simulink model "FullCardioLabModel"  (R2023b)
settings: Solver=FixedStepDiscrete  StartTime=0.0  StopTime=param_sim_time  FixedStep=1/fs  MaxStep=1/fs  RelTol=1e-3
undefined symbols (not defined in the file): analyses, fdesignblkfcn, fs, gcbh, param_tot_samples
libraries: dspstat3 x13, SCGAnalysis_SignalGenerationLib x2
(part 13 of 20)

== matlab function FullCardioLabModel/SCG Analysis/Enabled SCG Analysis Subsystem/Cardiac Interval Identification/Systolic Fiducial Point Marker/3D Systolic Fiducial Point Identifier ==
  data: fs input size=[1]; MC output size=[4*ceil(param_sim_time) 1]; MC_prelim input; IM_prelim input; IM output size=[4*ceil(param_sim_time) 1]; AO output size=[4*ceil(param_sim_time) 1]; AO_prelim input; scg_s1_3DMod input
function [MC, IM, AO] = slk_3D_systolic_fiducial_point_identifier(fs, MC_prelim, IM_prelim, AO_prelim, scg_s1_3DMod)
% Function to identify the (final) systolic hemodynamic fiducial points of the seismocardiogram (SCG) based on the preliminary systolic markers and using an S1 3D modulus signal.

% INPUTS:
% fs - the sampling frequency (in Hz).
% MC_prelim - preliminary sample indexes of mitral closure.
% IM_prelim - preliminary sample indexes isovolumic moment.
% AO_prelim_ - preliminary sample indexes of aortic opening.
% scg_s1_3DMod - the systolic (i.e, constructed from the S1 bandwidth-optimized x,y,z SCG components) 3DModulus signal.

% OUTPUTS:
% MC - final sample indexes of mitral closure.
% IM - final sample indexes isovolumic moment.
% AO - final sample indexes of aortic opening.

coder.extrinsic('legend');

% Plotting before refining.
Labelled3DSCG = figure;
plot(scg_s1_3DMod); hold on;
plot(IM_prelim, scg_s1_3DMod(IM_prelim),'xr')
plot(MC_prelim, scg_s1_3DMod(MC_prelim),'xb')
plot(AO_prelim, scg_s1_3DMod(AO_prelim),'xk')
box off

title('Systolic Fiducial Markers')
xlabel('Sample no.')
ylabel('Acceleration (mg)')

IM = zeros(length(IM_prelim), 1);   % Pre-initalization for speed.
MC = zeros(length(MC_prelim), 1);
AO = zeros(length(AO_prelim), 1);

MC_search_window_size = fs*0.02; % The window centered about MC_prelim where we will search for MC in the 3D Mod signal.
IM_search_window_size = fs*0.02; % The window centered about MC_prelim where we will search for MC in the 3D Mod signal.
AO_search_window_size = fs*0.04; % The window centered about MC_prelim where we will search for MC in the 3D Mod signal.


% Refining MC
for i = 1:length(MC_prelim)
    
    MC_search_window = scg_s1_3DMod(MC_prelim(i) - floor(MC_search_window_size/2):MC_prelim(i) + ceil(MC_search_window_size/2));
    [MC_candies_amps, MC_candies_locs, MC_candies_widths, MC_candies_proms]  = findpeaks(MC_search_window); % Identifying the amplitude, location, width, and prominence of the detected peaks.
    
    if MC_candies_amps % If peaks were detected...
        %MC_candy = MC_candies_locs(find(MC_candies_amps == max(MC_candies_amps))); % Consider MC as the peak with the maximum amplitude.
        %MC_candy = MC_candies_locs(1); % Consider MC as the first peak
        %MC_candy = MC_candies_locs(find(MC_candies_widths == max(MC_candies_widths))); % Consider MC as the peak with the greatest width.
        MC_candy = MC_candies_locs(find(MC_candies_proms == max(MC_candies_proms))); % Consider MC as the peak with the maximum prominence.
        MC(i) = -1 + MC_prelim(i) - floor(MC_search_window_size/2) + MC_candy;
    else
        MC(i) = nan;
    end
    
    MC_candy = []; % Clearing.
    MC_candies_amps = [];
    MC_candies_locs = [];
    MC_candies_widths = [];
    MC_candies_proms = [];
    
end

% Refining IM
for i = 1:length(IM_prelim)
    
    IM_search_window = scg_s1_3DMod(IM_prelim(i) - floor(IM_search_window_size/2):IM_prelim(i) + ceil(IM_search_window_size/2));
    [IM_candies_amps, IM_candies_locs, IM_candies_widths, IM_candies_proms]  = findpeaks(IM_search_window); % Identifying the amplitude, location, width, and prominence of the detected peaks.
    
    if IM_candies_amps % If peaks were detected...
        %IM_candy = IM_candies_locs(find(IM_candies_amps == max(IM_candies_amps))); % Consider IM as the peak with the maximum amplitude.
        %IM_candy = IM_candies_locs(1); % Consider IM as the first peak
        %IM_candy = IM_candies_locs(find(IM_candies_widths == max(IM_candies_widths))); % Consider IM as the peak with the greatest width.
        IM_candy = IM_candies_locs(find(IM_candies_proms == max(IM_candies_proms))); % Consider IM as the peak with the maximum prominence.
        IM(i) = -1 + IM_prelim(i) - floor(IM_search_window_size/2) + IM_candy;
    else
        IM(i) = nan;
    end
    
    IM_candy = []; % Clearing.
    IM_candies_amps = [];
    IM_candies_locs = [];
    IM_candies_widths = [];
    IM_candies_proms = [];
    
end

% Refining AO
for i = 1:length(AO_prelim)
    
    AO_lower_search_lim = max([IM(i), AO_prelim(i) - floor(AO_search_window_size/2)]); % Making sure the serach window does not include the IM peak.
    
    AO_search_window = scg_s1_3DMod(AO_lower_search_lim : AO_prelim(i) + ceil(AO_search_window_size/2));
    [AO_candies_amps, AO_candies_locs, AO_candies_widths, AO_candies_proms]  = findpeaks(AO_search_window); % Identifying the amplitude, location, width, and prominence of the detected peaks.
    
    if AO_candies_amps % If peaks were detected...
        %AO(i) = AO_candies_locs(find(AO_candies_amps == max(AO_candies_amps))); % Consider AO as the peak with the maximum amplitude.
        AO_candy = AO_candies_locs(1); % Consider AO as the first peak
        %AO_candy = AO_candies_locs(find(AO_candies_widths == max(AO_candies_widths))); % Consider AO as the peak with the greatest width.
        %AO_candy = AO_candies_locs(find(AO_candies_proms == max(AO_candies_proms))); % Consider AO as the peak with the maximum prominence.
        AO(i) = -1 + AO_lower_search_lim + AO_candy;
    else
        AO(i) = nan;
    end
    
    AO_candy = []; % Clearing.
    AO_candies_amps = [];
    AO_candies_locs = [];
    AO_candies_widths = [];
    AO_candies_proms = [];
    AO_lower_search_lim = [];
    
end

figure(Labelled3DSCG);
hold on;
plot(IM(~isnan(IM)), scg_s1_3DMod(IM(~isnan(IM))),'or') % Do not plot the 'nans'.
plot(MC(~isnan(MC)), scg_s1_3DMod(MC(~isnan(MC))),'ob')
plot(AO(~isnan(AO)), scg_s1_3DMod(AO(~isnan(AO))),'ok')

legend('3D Modulus','IM_p_r_e_l_i_m','MC_p_r_e_l_i_m','AO_p_r_e_l_i_m','IM','MC','AO')

end

== matlab function FullCardioLabModel/SCG Analysis/Enabled SCG Analysis Subsystem/Cardiac Interval Identification/Diastolic Fiducial Point Marker/3D Diastolic Fiducial Point Identifier ==
  data: fs input size=[1]; AC output size=[4*ceil(param_sim_time) 1]; AC_prelim input; MO_prelim input; MO output size=[4*ceil(param_sim_time) 1]; scg_s2_3DMod input
function [AC, MO] = slk_3D_diastolic_fiducial_point_identifier(fs, AC_prelim, MO_prelim, scg_s2_3DMod)
% Function to identify the (final) diastolic hemodynamic fiducial points of the seismocardiogram (SCG) based on the preliminary diastolic markers and using an S2 3D modulus signal.

% INPUTS:
% fs - the sampling frequency (in Hz).
% AC_prelim - preliminary sample indexes of aortic closure.
% MO_prelim - preliminary sample indexes mitral opening.
% scg_s2_3DMod - the diastolic (i.e, constructed from the S2 bandwidth-optimized x,y,z SCG components) 3DModulus signal.

% OUTPUTS:
% AC - final sample indexes of aortic opening.
% MO - final sample indexes of mitral opening.

coder.extrinsic('legend');

% Plotting before refining.
Labelled3DSCG = figure;
plot(scg_s2_3DMod); hold on;
plot(AC_prelim(~isnan(AC_prelim)), scg_s2_3DMod(AC_prelim(~isnan(AC_prelim))),'xb') % Do not plot the 'nans'.
plot(MO_prelim(~isnan(MO_prelim)), scg_s2_3DMod(MO_prelim(~isnan(MO_prelim))),'xr')
box off

title('Diastolic Fiducial Markers')
xlabel('Sample no.')
ylabel('Acceleration (mg)')

AC = zeros(length(MO_prelim), 1);   % Pre-initalization for speed.
MO = zeros(length(AC_prelim), 1);


AC_search_window_size = fs*0.02; % The window centered about AC_prelim where we will search for AC in the 3D Mod signal.
MO_search_window_size = fs*0.02; % The window centered about MO_prelim where we will search for MO in the 3D Mod signal.


% Refining AC
for i = 1:length(AC_prelim)
    
    if isnan(AC_prelim(i))
        
        AC(i) = nan;

    else
        
        AC_search_window = scg_s2_3DMod(AC_prelim(i) - floor(AC_search_window_size/2):AC_prelim(i) + ceil(AC_search_window_size/2));
        [AC_candies_amps, AC_candies_locs, AC_candies_widths, AC_candies_proms]  = findpeaks(AC_search_window); % Identifying the amplitude, location, width, and prominence of the detected peaks.
        
        if AC_candies_amps % If peaks were detected...
            %AC_candy = MC_candies_locs(find(MC_candies_amps == max(MC_candies_amps)));      % Consider AC as the peak with the maximum amplitude.
            %AC_candy = MC_candies_locs(1);                                                  % Consider AC as the first peak.
            %AC_candy = MC_candies_locs(find(MC_candies_widths == max(MC_candies_widths)));  % Consider AC as the peak with the greatest width.
            AC_candy = AC_candies_locs(find(AC_candies_proms == max(AC_candies_proms)));     % Consider AC as the peak with the maximum prominence.
            AC(i) = -1 + AC_prelim(i) - floor(AC_search_window_size/2) + AC_candy;
        else
            AC(i) = nan;
        end
        
        AC_candy = []; % Clearing.
        AC_candies_amps = [];
        AC_candies_locs = [];
        AC_candies_widths = [];
        AC_candies_proms = [];
        
    end
end

% Refining MO
for i = 1:length(MO_prelim)
    
    if isnan(MO_prelim(i))
        
        MO(i) = nan;
        
    else
        
        MO_search_window = scg_s2_3DMod(MO_prelim(i) - floor(MO_search_window_size/2):MO_prelim(i) + ceil(MO_search_window_size/2));
        [MO_candies_amps, MO_candies_locs, MO_candies_widths, MO_candies_proms]  = findpeaks(MO_search_window); % Identifying the amplitude, location, width, and prominence of the detected peaks.
        
        if MO_candies_amps % If peaks were detected...
            %MO_candy = IM_candies_locs(find(MO_candies_amps == max(MO_candies_amps)));       % Consider MO as the peak with the maximum amplitude.
            %MO_candy = IM_candies_locs(1);                                                   % Consider MO as the first peak
            %MO_candy = IM_candies_locs(find(IM_candies_widths == max(IM_candies_widths)));   % Consider MO as the peak with the greatest width.
            MO_candy = MO_candies_locs(find(MO_candies_proms == max(MO_candies_proms)));     % Consider MO as the peak with the maximum prominence.
            MO(i) = -1 + MO_prelim(i) - floor(MO_search_window_size/2) + MO_candy;
        else
            AC(i) = nan;
        end
        
        MO_candy = []; % Clearing.
        MO_candies_amps = [];
        MO_candies_locs = [];
        MO_candies_widths = [];
        MO_candies_proms = [];
        
    end
    
end

figure(Labelled3DSCG);
hold on;
plot(AC(~isnan(AC)), scg_s2_3DMod(AC(~isnan(AC))),'ob') % Do not plot the 'nans'.
plot(MO(~isnan(MO)), scg_s2_3DMod(MO(~isnan(MO))),'or')

legend('3D Modulus','AC_p_r_e_l_i_m','MO_p_r_e_l_i_m','AC','MO')

end

== matlab function FullCardioLabModel/SCG Analysis/Enabled SCG Analysis Subsystem/Cardiac Interval Identification/Diastolic Fiducial Point Marker/Preliminary Diastolic Fiducial Point Identifier ==
  data: fs input size=[1]; AC_prelim output size=[4*ceil(param_sim_time) 1]; idx_r input; idx_t input; MO_prelim output size=[4*ceil(param_sim_time) 1]; scg_s2_ref_signal input
function [AC_prelim, MO_prelim] = slk_preliminary_diastolic_fiducial_point_identifier(fs, idx_r, idx_t, scg_s2_ref_signal)
% Function to identify the preliminary diastolic hemodynamic fiducial points of the seismocardiogram (SCG) using an S2 reference signal.

% INPUTS:
% fs - Sampling frequency (Hz).
% idx_r - ECG R peak indexes.
% idx_t - ECG T peak indexes.
% scg_s2_ref_signal - SCG diastolic reference signal.

% OUTPUTS:
% AC_prelim - Preliminary sample indexes of aortic closure.
% MO_prelim - Preliminary sample indexes of mitral opening.

% Ensure idx_t and idx_r are coherent in size
if ~isempty(idx_t) && length(idx_r) ~= length(idx_t)
    error('idx_r and idx_t must have the same length if idx_t is provided.');
end

num_cycles = length(idx_r) - 1; % Exclude the last cycle - high risk of diastolic fiducial points being cut-off.
AC_prelim = nan(num_cycles, 1); % Pre-allocate outputs.
MO_prelim = nan(num_cycles, 1);

rr_intervals = diff(idx_r); % RR intervals.

% Window limits (relative to RR interval or absolute values).
if isempty(idx_t)
    s2_1st_search_window_relative_lims = [0.2, 0.9];
else
    s2_1st_search_window_relative_lims = [-0.075, 0.9];
end
s2_2nd_search_window_lims = [-0.025*fs, 0.0125*fs];
AC_prelim_window_lims = [-0.015*fs, 0];
MO_prelim_window_lims = [0, 0.1*fs];

% Iterating through cycles
for i = 1:num_cycles
    cycle_start = idx_r(i);
    cycle_end = idx_r(i + 1);
    cycle = scg_s2_ref_signal(cycle_start:cycle_end);
    rr_interval = rr_intervals(i);

    % Compute TKEO of the cycle
    tkeo_cycle = tkeo(cycle);

    % Define the 1st anchor search window
    if isempty(idx_t) || isnan(idx_t(i))
        first_window_start = floor(rr_interval*s2_1st_search_window_relative_lims(1));
        first_window_end   = ceil(rr_interval*s2_1st_search_window_relative_lims(2));
    else
        t_peak_rel = idx_t(i) - cycle_start;
        first_window_start = t_peak_rel + floor(rr_interval*s2_1st_search_window_relative_lims(1));
        first_window_end = ceil(rr_interval*s2_1st_search_window_relative_lims(2));
    end

    % Ensure window indices are within bounds
    first_window_start = max(1, first_window_start);
    first_window_end = min(length(tkeo_cycle), first_window_end);

    % First anchor (S2 peak in TKEO)
    [~, locs, ~, proms] = findpeaks(tkeo_cycle(first_window_start:first_window_end));
    if isempty(proms), continue; end % Skip if no peaks found.
    [~, max_idx] = max(proms);
    s2_1st_anchor = first_window_start + locs(max_idx) - 1;

    % Second anchor (S2 trough in original signal)
    second_window_start = max(1, round(s2_1st_anchor + s2_2nd_search_window_lims(1)));
    second_window_end = min(length(cycle), round(s2_1st_anchor + s2_2nd_search_window_lims(2)));
    [~, locs, ~, ~] = findpeaks(-cycle(second_window_start:second_window_end));
    if isempty(locs), continue; end % Skip if no troughs found
    [~, min_idx] = max(-cycle(second_window_start + locs - 1));
    s2_2nd_anchor = second_window_start + locs(min_idx) - 1;

    % AC_prelim (peak before 2nd anchor)
    ac_window_start = max(1, s2_2nd_anchor + AC_prelim_window_lims(1));
    ac_window_end = max(ac_window_start, min(length(cycle), s2_2nd_anchor + AC_prelim_window_lims(2)));
    [~, locs] = findpeaks(cycle(ac_window_start:ac_window_end));
    if ~isempty(locs)
        AC_prelim(i) = cycle_start + ac_window_start + locs(end) - 1; % Last peak before the 2nd anchor
    end

    % MO_prelim (trough after 2nd anchor)
    mo_window_start = max(1, s2_2nd_anchor + MO_prelim_window_lims(1));
    mo_window_end = min(length(cycle), s2_2nd_anchor + MO_prelim_window_lims(2));
    [~, locs, ~, proms] = findpeaks(-cycle(mo_window_start:mo_window_end));
    if ~isempty(proms)
        [~, max_idx] = max(proms);
        MO_prelim(i) = cycle_start + mo_window_start + locs(max_idx) - 1;
    end
end

% Plot results
t = (0:length(scg_s2_ref_signal) - 1) / fs;
figure;
plot(t, scg_s2_ref_signal); hold on;
plot((AC_prelim(~isnan(AC_prelim)) - 1) / fs, scg_s2_ref_signal(AC_prelim(~isnan(AC_prelim))), 'or');
plot((MO_prelim(~isnan(MO_prelim)) - 1) / fs, scg_s2_ref_signal(MO_prelim(~isnan(MO_prelim))), 'ob');
legend('SCG S2 Reference Signal', 'AC\_prelim', 'MO\_prelim');
title('Preliminary Diastolic Fiducial Markers');
xlabel('Time (sec)');
ylabel('Amplitude');
box off;

end

== matlab function FullCardioLabModel/SCG Analysis/Enabled SCG Analysis Subsystem/Cardiac Interval Identification/Average Calculator/slk_average_calculator ==
  data: average_type input size=[1]; series input; average output size=[1]
function average = slk_average_calculator(average_type, series)
% Simple function to return the user-defined average of an input series.

average = 0; % Pre-initialization

if average_type == 1
    average = mean(series(~isnan(series)));
elseif average_type == 2
    average = median(series(~isnan(series)));
elseif average_type == 3
    average = mode(series(~isnan(series)));
end

end

== matlab function FullCardioLabModel/SCG Analysis/Enabled SCG Analysis Subsystem/Cardiac Interval Identification/MATLAB Function ==
  data: PEP output size=[4*ceil(param_sim_time) 1]; fs input size=[1]; IVC output size=[4*ceil(param_sim_time) 1]; ecg_q input; ecg_r input; ecg_t input; MC input; AO input; AC input; MO input; ET output size=[4*ceil(param_sim_time) 1]; IVR output size=[4*ceil(param_sim_time) 1]; DC output size=[4*ceil(param_sim_time) 1]
function [PEP, IVC, ET, IVR, DC]  = slk_cardiac_interval_identifier(fs, ecg_q, ecg_r, ecg_t, MC, AO, AC, MO)
% Function to calculate various cardiac intervals based on the previously-identified systolic and diastolic fiducial markers.

% INPUTS
% fs = sampling frequency.
% ecg_q = Q peak indices of the ECG.
% ecg_r = R peak indices of the ECG.
% MC = Mitral Closure indices of the SCG.
% IM = Isovolumic Moment indices of the SCG.
% AO = Aortic Opening indices of the SCG.
% MC = Mitral Closure indices of the SCG.

% OUTPUTS
% PEP = Pre-Ejection Period indices.
% IVC = Isovolumic Contraction indices.
% EJ = Ejection Time indices.
% IVR = Isovolumic Relaxation indices.

num_cycles = length(ecg_r) - 1; % Remember, the last cycle was not considered for systolic and diastolic fiducial point identification. 

IVC = zeros(num_cycles, 1); % Pre-initialization for speed.
PEP = zeros(num_cycles, 1);
ET = zeros(num_cycles, 1);
IVR = zeros(num_cycles, 1);
DC = zeros(num_cycles, 1);

for i = 2:num_cycles % We also don't consider the first cycle because there are often misdetections in the Q complex.
    
    %PEP (AO - Q or AO - R).
    if ecg_q(i) && ~isnan(AO(i))
        PEP(i) = (AO(i) - ecg_q(i))/fs;
    elseif ecg_r(i) && ~isnan(AO(i))
        PEP(i) = (AO(i) - ecg_q(i))/fs;
    else
        PEP(i) = nan;
    end
        
    %IVC (AO - MC).
    if ~isnan(MC(i)) && ~isnan(AO(i))
        IVC(i) = (AO(i) - MC(i))/fs;
    else
        IVC(i) = nan;
    end
    
    %ET (AC - AO).
    if ~isnan(AC(i)) && ~isnan(AO(i))
        ET(i) = (AC(i) - AO(i))/fs;
    else
        ET(i) = nan;
    end
    
    %IVR (MO - AC).
    if ~isnan(MO(i)) && ~isnan(AC(i))
        IVR(i) = (MO(i) - AC(i))/fs;
    else
        IVR(i) = nan;
    end
    
    % DC (T - AC) - In healthy cases, should be negative! If positive - there is diastolic contraction!
    if ~isnan(ecg_t(i)) && ~isnan(AC(i))
        DC(i) = (ecg_t(i) - AC(i))/fs;
    else
        DC(i) = nan;
    end
    
end

IVC(1) = []; % Deleting the non-calculated first cycle (which was initialized to 0).
PEP(1) = []; 
ET(1) = []; 
IVR(1) = []; 
DC(1) = []; 
end

== matlab function FullCardioLabModel/SCG Analysis/Enabled SCG Analysis Subsystem/Cardiac Interval Identification/Average Calculator1/slk_average_calculator ==
  data: average_type input size=[1]; series input; average output size=[1]
function average = slk_average_calculator(average_type, series)
% Simple function to return the user-defined average of an input series.

average = 0; % Pre-initialization

if average_type == 1
    average = mean(series(~isnan(series)));
elseif average_type == 2
    average = median(series(~isnan(series)));
elseif average_type == 3
    average = mode(series(~isnan(series)));
end

end

== matlab function FullCardioLabModel/ECG Analysis/Enabled ECG Analysis Subsystem/Assign To Workspace: Num Cycles/Enabled To Workspace ECG Num Cycles/Slk Wrapped Assigned To Workspace ==
  data: assigned_var input size=[1]
function slk_wrapped_assign_to_workspace(assigned_var)
% Wrapped simulink function to assign an input 'assigned_var' to the base workspace.

coder.extrinsic('assign_num_cycles_to_workspace');

if assigned_var % Only go into the function if a valid variable is passed to it.
    assign_num_cycles_to_workspace(assigned_var)
end

end

== matlab function FullCardioLabModel/SCG Analysis/Enabled SCG Analysis Subsystem/Cardiac Interval Identification/Average Calculator2/slk_average_calculator ==
  data: average_type input size=[1]; series input; average output size=[1]
function average = slk_average_calculator(average_type, series)
% Simple function to return the user-defined average of an input series.

average = 0; % Pre-initialization

if average_type == 1
    average = mean(series(~isnan(series)));
elseif average_type == 2
    average = median(series(~isnan(series)));
elseif average_type == 3
    average = mode(series(~isnan(series)));
end

end

== matlab function FullCardioLabModel/SCG Analysis/Enabled SCG Analysis Subsystem/Cardiac Interval Identification/Average Calculator3/slk_average_calculator ==
  data: average_type input size=[1]; series input; average output size=[1]
function average = slk_average_calculator(average_type, series)
% Simple function to return the user-defined average of an input series.

average = 0; % Pre-initialization

if average_type == 1
    average = mean(series(~isnan(series)));
elseif average_type == 2
    average = median(series(~isnan(series)));
elseif average_type == 3
    average = mode(series(~isnan(series)));
end

end

== matlab function FullCardioLabModel/SCG Analysis/Enabled SCG Analysis Subsystem/Cardiac Interval Identification/Average Calculator4/slk_average_calculator ==
  data: average_type input size=[1]; series input; average output size=[1]
function average = slk_average_calculator(average_type, series)
% Simple function to return the user-defined average of an input series.

average = 0; % Pre-initialization

if average_type == 1
    average = mean(series(~isnan(series)));
elseif average_type == 2
    average = median(series(~isnan(series)));
elseif average_type == 3
    average = mode(series(~isnan(series)));
end

end

== matlab function FullCardioLabModel/ECG Analysis/Enabled ECG Analysis Subsystem/Assign To Workspace: idxs PQRST/Enabled To Workspace idxs PQRST/Slk Wrapped Assigned to Workspace ==
  data: idxs_pqrst input size=[4*ceil(param_sim_time) 5]
function slk_wrapped_assign_to_workspace(idxs_pqrst)
% Wrapped simulink function to assign an input 'assigned_var' to the base workspace.

coder.extrinsic('assign_idxs_pqrst_to_workspace');

if idxs_pqrst(:,3) % Only go into the function if a valid ECG R pos sequence is passed to it.
    assign_idxs_pqrst_to_workspace(idxs_pqrst);
end

end

== matlab function FullCardioLabModel/SCG Analysis/Enabled SCG Analysis Subsystem/Signal Generation/3D Projections/SCG xyz Average Cycle/Average SCGxyz Cycle Calculator ==
  data: r_pos input; scgxyz input; scgxyz_avgcycle output size=[3*fs 3]
function scgxyz_avgcycle  = slk_avg_scgxyz_cycle_calculator(r_pos,scgxyz)
% Simulink function to return the average x,y, and z cycles of the SCG.

% INPUTS:
% r_pos = index positions of the R peaks of the ecg.
% scgxyz = matrix of size [length_scg 3] with the (normally pre-processed) SCG
%          x,y, and z components. The first column corresponds to SCGx, the second
%          to SCGy and the third to SCGz.

% OUTPUT:
% avg_scg_xyz = matrix of size [min_rr 3] with the average SCG cycles of
%               the x,y, and z components. The first column corresponds to SCGx, the second
%               to SCGy and the third to SCGz 


% Calculating number of cycles to be considered in averaging (considered_cycles).
rr_min = min(diff(r_pos)); % Shortest cycle length - all the cycles will but cut down to this length.

if length(scgxyz) > r_pos(end) + rr_min
    considered_cycles = length(r_pos);
else
    considered_cycles = length(r_pos) - 1;
end

scg_x_cycles = zeros(rr_min,considered_cycles);
scg_y_cycles = zeros(rr_min,considered_cycles);
scg_z_cycles = zeros(rr_min,considered_cycles);

fig_scg_average_cycles = figure;

% Isolating and plotting each cycle
for i = 1:considered_cycles
    figure(fig_scg_average_cycles);
    scg_x_cycles(:,i) = scgxyz(r_pos(i):r_pos(i) + rr_min - 1,1);
    scg_y_cycles(:,i) = scgxyz(r_pos(i):r_pos(i) + rr_min - 1,2);
    scg_z_cycles(:,i) = scgxyz(r_pos(i):r_pos(i) + rr_min - 1,3);
    
    % Plotting
    subplot(3,1,1); plot(scg_x_cycles(:,i),'b'); hold on;
    subplot(3,1,2); plot(scg_y_cycles(:,i),'b'); hold on;
    subplot(3,1,3); plot(scg_z_cycles(:,i),'b'); hold on;
end

% Calculating average cycle
avg_scg_x = mean(scg_x_cycles,2);
avg_scg_y = mean(scg_y_cycles,2);
avg_scg_z = mean(scg_z_cycles,2);

% Plotting the average cycle
subplot(3,1,1); plot(avg_scg_x,'k','LineWidth',2); title('Average SCG x'); box off;
subplot(3,1,2); plot(avg_scg_y,'k','LineWidth',2); title('Average SCG y'); ylabel('Amplitude (mg)'); box off;
subplot(3,1,3); plot(avg_scg_z,'k','LineWidth',2); title('Average SCG z'); xlabel('Time (msec)'); box off;

scgxyz_avgcycle = [avg_scg_x avg_scg_y avg_scg_z];
end

== matlab function FullCardioLabModel/SCG Analysis/Enabled SCG Analysis Subsystem/Signal Generation/3D Projections/SCG xyz Average Cycle/Min RR Calculator ==
  data: r_pos input; min_rr output size=[1]
function min_rr  = slk_min_rr_calculator(r_pos)
% Simulink function to calculate the shortest RR interval from a sequence
% of R peak inputs.

% INPUTS:
% r_pos = index positions of the R peaks of the ecg.

% OUTPUT:
% min_rr = minimum RR interval.

if r_pos % Only enter the function if a valid r_pos sequence is passed to it.
    min_rr = min(diff(r_pos)); % Shortest cycle length - all the cycles will but cut down to this length.
else
    min_rr = 0;
end
end

== matlab function FullCardioLabModel/SCG Analysis/Enabled SCG Analysis Subsystem/3D Anisotropy Characterization/Average Cycle Max Diameter//Volume Calculator/Wrapped Average Cycle Max Diameter//Volume Calculator ==
  data: avg_s1_xyz input size=[0.2*fs 3]; avg_cycle_max_diameter_over_volume output size=[1]
function avg_cycle_max_diameter_over_volume = wrapped_anisotropy_calculator_avg_cycle_max_diameter_over_vol(avg_s1_xyz) 
avg_cycle_max_diameter_over_volume = -1; % Pre-Initialization.
coder.extrinsic('anisotropy_calculator_avg_cycle_max_diameter_over_volume');
avg_cycle_max_diameter_over_volume = anisotropy_calculator_avg_cycle_max_diameter_over_volume(avg_s1_xyz); 
end

== matlab function FullCardioLabModel/SCG Analysis/Enabled SCG Analysis Subsystem/3D Anisotropy Characterization/Average Cycle Max Diameter//Volume Calculator/SCG xyz Average Cycle/Average SCGxyz Cycle Calculator ==
  data: r_pos input; scgxyz input; scgxyz_avgcycle output size=[3*fs 3]
function scgxyz_avgcycle  = slk_avg_scgxyz_cycle_calculator(r_pos,scgxyz)
% Simulink function to return the average x,y, and z cycles of the SCG.

% INPUTS:
% r_pos = index positions of the R peaks of the ecg.
% scgxyz = matrix of size [length_scg 3] with the (normally pre-processed) SCG
%          x,y, and z components. The first column corresponds to SCGx, the second
%          to SCGy and the third to SCGz.

% OUTPUT:
% avg_scg_xyz = matrix of size [min_rr 3] with the average SCG cycles of
%               the x,y, and z components. The first column corresponds to SCGx, the second
%               to SCGy and the third to SCGz 


% Calculating number of cycles to be considered in averaging (considered_cycles).
rr_min = min(diff(r_pos)); % Shortest cycle length - all the cycles will but cut down to this length.

if length(scgxyz) > r_pos(end) + rr_min
    considered_cycles = length(r_pos);
else
    considered_cycles = length(r_pos) - 1;
end

scg_x_cycles = zeros(rr_min,considered_cycles);
scg_y_cycles = zeros(rr_min,considered_cycles);
scg_z_cycles = zeros(rr_min,considered_cycles);

% fig_scg_average_cycles = figure;

% Isolating and plotting each cycle
for i = 1:considered_cycles
%     figure(fig_scg_average_cycles);
    scg_x_cycles(:,i) = scgxyz(r_pos(i):r_pos(i) + rr_min - 1,1);
    scg_y_cycles(:,i) = scgxyz(r_pos(i):r_pos(i) + rr_min - 1,2);
    scg_z_cycles(:,i) = scgxyz(r_pos(i):r_pos(i) + rr_min - 1,3);
    
    % Plotting
%     subplot(3,1,1); plot(scg_x_cycles(:,i),'b'); hold on;
%     subplot(3,1,2); plot(scg_y_cycles(:,i),'b'); hold on;
%     subplot(3,1,3); plot(scg_z_cycles(:,i),'b'); hold on;
end

% Calculating average cycle
avg_scg_x = mean(scg_x_cycles,2);
avg_scg_y = mean(scg_y_cycles,2);
avg_scg_z = mean(scg_z_cycles,2);

% Plotting the average cycle
% subplot(3,1,1); plot(avg_scg_x,'k','LineWidth',2); title('Average SCG x'); box off;
% subplot(3,1,2); plot(avg_scg_y,'k','LineWidth',2); title('Average SCG y'); ylabel('Amplitude (mg)'); box off;
% subplot(3,1,3); plot(avg_scg_z,'k','LineWidth',2); title('Average SCG z'); xlabel('Time (msec)'); box off;

scgxyz_avgcycle = [avg_scg_x avg_scg_y avg_scg_z];
end

== matlab function FullCardioLabModel/SCG Analysis/Enabled SCG Analysis Subsystem/3D Anisotropy Characterization/Average Cycle Max Diameter//Volume Calculator/SCG xyz Average Cycle/Min RR Calculator ==
  data: r_pos input; min_rr output size=[1]
function min_rr  = slk_min_rr_calculator(r_pos)
% Simulink function to calculate the shortest RR interval from a sequence
% of R peak inputs.

% INPUTS:
% r_pos = index positions of the R peaks of the ecg.

% OUTPUT:
% min_rr = minimum RR interval.

if r_pos % Only enter the function if a valid r_pos sequence is passed to it.
    min_rr = min(diff(r_pos)); % Shortest cycle length - all the cycles will but cut down to this length.
else
    min_rr = 0;
end
end

== matlab function FullCardioLabModel/SCG Analysis/Enabled SCG Analysis Subsystem/3D Anisotropy Characterization/Average Cycle Max//Median Diameter Calculator/SCG xyz Average Cycle/Average SCGxyz Cycle Calculator ==
  data: r_pos input; scgxyz input; scgxyz_avgcycle output size=[3*fs 3]
function scgxyz_avgcycle  = slk_avg_scgxyz_cycle_calculator(r_pos,scgxyz)
% Simulink function to return the average x,y, and z cycles of the SCG.

% INPUTS:
% r_pos = index positions of the R peaks of the ecg.
% scgxyz = matrix of size [length_scg 3] with the (normally pre-processed) SCG
%          x,y, and z components. The first column corresponds to SCGx, the second
%          to SCGy and the third to SCGz.

% OUTPUT:
% avg_scg_xyz = matrix of size [min_rr 3] with the average SCG cycles of
%               the x,y, and z components. The first column corresponds to SCGx, the second
%               to SCGy and the third to SCGz 


% Calculating number of cycles to be considered in averaging (considered_cycles).
rr_min = min(diff(r_pos)); % Shortest cycle length - all the cycles will but cut down to this length.

if length(scgxyz) > r_pos(end) + rr_min
    considered_cycles = length(r_pos);
else
    considered_cycles = length(r_pos) - 1;
end

scg_x_cycles = zeros(rr_min,considered_cycles);
scg_y_cycles = zeros(rr_min,considered_cycles);
scg_z_cycles = zeros(rr_min,considered_cycles);

% fig_scg_average_cycles = figure;

% Isolating and plotting each cycle
for i = 1:considered_cycles
%     figure(fig_scg_average_cycles);
    scg_x_cycles(:,i) = scgxyz(r_pos(i):r_pos(i) + rr_min - 1,1);
    scg_y_cycles(:,i) = scgxyz(r_pos(i):r_pos(i) + rr_min - 1,2);
    scg_z_cycles(:,i) = scgxyz(r_pos(i):r_pos(i) + rr_min - 1,3);
    
    % Plotting
%     subplot(3,1,1); plot(scg_x_cycles(:,i),'b'); hold on;
%     subplot(3,1,2); plot(scg_y_cycles(:,i),'b'); hold on;
%     subplot(3,1,3); plot(scg_z_cycles(:,i),'b'); hold on;
end

% Calculating average cycle
avg_scg_x = mean(scg_x_cycles,2);
avg_scg_y = mean(scg_y_cycles,2);
avg_scg_z = mean(scg_z_cycles,2);

% Plotting the average cycle
% subplot(3,1,1); plot(avg_scg_x,'k','LineWidth',2); title('Average SCG x'); box off;
% subplot(3,1,2); plot(avg_scg_y,'k','LineWidth',2); title('Average SCG y'); ylabel('Amplitude (mg)'); box off;
% subplot(3,1,3); plot(avg_scg_z,'k','LineWidth',2); title('Average SCG z'); xlabel('Time (msec)'); box off;

scgxyz_avgcycle = [avg_scg_x avg_scg_y avg_scg_z];
end

== matlab function FullCardioLabModel/SCG Analysis/Enabled SCG Analysis Subsystem/3D Anisotropy Characterization/Average Cycle Max//Median Diameter Calculator/SCG xyz Average Cycle/Min RR Calculator ==
  data: r_pos input; min_rr output size=[1]
function min_rr  = slk_min_rr_calculator(r_pos)
% Simulink function to calculate the shortest RR interval from a sequence
% of R peak inputs.

% INPUTS:
% r_pos = index positions of the R peaks of the ecg.

% OUTPUT:
% min_rr = minimum RR interval.

if r_pos % Only enter the function if a valid r_pos sequence is passed to it.
    min_rr = min(diff(r_pos)); % Shortest cycle length - all the cycles will but cut down to this length.
else
    min_rr = 0;
end
end

== matlab function FullCardioLabModel/SCG Analysis/Enabled SCG Analysis Subsystem/3D Anisotropy Characterization/Average Cycle Max//Median Diameter Calculator/Wrapped Average Cycle Max//Median Diameter Calculator ==
  data: avg_s1_xyz input size=[0.2*fs 3]; avg_cycle_max_over_median_diameter output size=[1]
function avg_cycle_max_over_median_diameter = wrapped_anisotropy_calculator_avg_cycle_max_over_med_diameter(avg_s1_xyz) 
avg_cycle_max_over_median_diameter = -1; % Pre-Initialization.
coder.extrinsic('anisotropy_calculator_avg_cycle_max_over_median_diameter');
avg_cycle_max_over_median_diameter = anisotropy_calculator_avg_cycle_max_over_median_diameter(avg_s1_xyz); 
end

== matlab function FullCardioLabModel/SCG Analysis/Enabled SCG Analysis Subsystem/All Signals Signal Metric Characterization/SCG X Signal Metric Characterization/Average S1 peak-to-peak Amplitude Calculator/Average S1p2p Amplitude Calculator ==
  data: fs input; r_pos input; scg_signal input; average_s1p2pamp output size=[1]
function average_s1p2pamp = slk_average_s1p2pamp_calculator(fs, r_pos, scg_signal)
% Function to calculate the average (mean) S1 peak-to-peak amplitude from an SCG input signal.

coder.extrinsic('sgtitle'); % Needed later for plotting.

num_cycles = length(r_pos);

s1p2pamp = zeros(1,num_cycles); % Pre-initialization for speed.
s1_peak_pos = zeros(1,num_cycles); 
s1_trough_pos = zeros(1,num_cycles); 
s1 = zeros(0.2*fs,1);

for i = 1:num_cycles 
    s1 = scg_signal(r_pos(i):r_pos(i) + 0.2*fs); % The S1 complex is considered as the 200ms following the R wave.
    s1_peak_pos(i) = r_pos(i) + find(s1 == max(s1));
    s1_trough_pos(i) = r_pos(i) + find(s1 == min(s1));
    s1p2pamp(i) = max(s1) - min(s1); % S1 peak-to-peak amplitude is the max minus the min inside the S1 window.   
end

average_s1p2pamp = mean(s1p2pamp);

%% Plotting.

figure;
sgtitle('SCG x')
ax = [0 0]; % Pre-initialization

% Labelled SCG.
t = 0:1/fs:(length(scg_signal)-1)/fs;

ax(1) = subplot(2,1,1);
plot(t,scg_signal); hold on
plot((s1_peak_pos-1)/fs, scg_signal(s1_peak_pos), 'ro') % Plotting the peaks.
plot((s1_trough_pos-1)/fs, scg_signal(s1_trough_pos), 'bo') % Plotting the troughs.
ylim([min(scg_signal)-10 max(scg_signal)+10]);

% Green Vertical Lines to Denote R peak Positions.
for i = 1:num_cycles
    plot([(r_pos(i) - 1)/fs (r_pos(i) - 1)/fs],[min(scg_signal)-10 max(scg_signal)+10],'g--')
end

title('Labelled S1 Peaks + Troughs')
xlabel('Time (sec)')
ylabel('Acceleration (mg)')
box off

%% S1 p2p Amplitude Evolution.
ax(2) = subplot(2,1,2);
plot((((s1_peak_pos + s1_trough_pos)/2)-1)/fs, s1p2pamp,'.-'); hold on % Plotting the S1 P2P Amp. at the timepoints given by the midpoint between the detected S1 peaks and troughs.
xlabel('Time (sec)')
ylabel('Peak-to-Peak Amplitude (mg)')
title('S1 P2P Amplitude Evolution');
plot([0 (r_pos(end)-1)/fs], [average_s1p2pamp average_s1p2pamp],'r--') % Plotting the average S1 P2P Amp.
box off

linkaxes(ax,'x')

end

== matlab function FullCardioLabModel/ECG Analysis/Enabled ECG Analysis Subsystem/Coherent Segmentation/Slk Coherent Segmentation Function ==
  data: idxs_p input size=[4*ceil(param_sim_time) 1]; idxs_coherent_pqrst output size=[4*ceil(param_sim_time) 5]; idxs_q input size=[4*ceil(param_sim_time) 1]; idxs_r input size=[4*ceil(param_sim_time) 1]; idxs_s input size=[4*ceil(param_sim_time) 1]; idxs_t input size=[4*ceil(param_sim_time) 1]; num_cycles output size=1
function [idxs_coherent_pqrst, num_cycles] = slk_coherent_segmentation(idxs_p, idxs_q, idxs_r, idxs_s, idxs_t)
% Function to associate the detected PQRST peaks to each other in a coherent way. 
% The function will produce an output 'idxs_coherent_pqrst' of size [num_cycles x 5], where the number of cycles is determined by the number of R peaks. The 5 corresponds to the 5 fiducial points (PQRST peaks).
% num_cycles is the number of detected R peaks (heart cycles). 
% The first column of coherent_prqst corresponds to the detected P waves (and so on for Q,R,S,T), where the row corresponds to that cycle number. 
% If a P wave was not detected for that cycle, it is replaced with 'Nan'.

% INPUTS:
% idxs_p/q/r/s/t (vector) - vectors of possibly different lengths (corresponding to the number of detected p/q/r/s/t peaks)

if idxs_r % Only go into the function if a valid ecg R peak sequence is passed to it (Simulink particularity).
    
    % Preinitialization.
    idxs_coherent_p = zeros(length(idxs_r),1);
    idxs_coherent_q = zeros(length(idxs_r),1);
    idxs_coherent_r = zeros(length(idxs_r),1);
    idxs_coherent_s = zeros(length(idxs_r),1);
    idxs_coherent_t = zeros(length(idxs_r),1);
        

    %% First Heart Cycle.
    
    % P Wave.
    temp = idxs_p(idxs_p < idxs_r(1));
    if isempty(temp) || temp(end) == 0
        idxs_coherent_p(1) = nan;
        temp = [];
    else
        idxs_coherent_p(1) = temp(end); % If more than 1 P waves are detected before the first R wave (rare), consider the one closest to the R peak.
    end
    
    % Q Wave.
    temp = idxs_p(idxs_q < idxs_r(1));
    if isempty(temp) || temp(end) == 0
        idxs_coherent_q(1) = nan;
        temp = [];
    else
        idxs_coherent_q(1) = temp(end); % If more than 1 Q waves are detected before the first R wave (rare), consider the one closest to the R peak.
    end
    
    % R Wave.
    idxs_coherent_r(1) = idxs_r(1); % R waves are always detected and are the easiest to detect. Therefore they are the fiducal points determining segmentation. 
    
    % S Wave.
    temp = idxs_s(idxs_s > idxs_r(1) & idxs_s < idxs_r(2));
    if isempty(temp)
        idxs_coherent_s(1) = nan;
        temp = [];
    else
        idxs_coherent_s(1) = temp(end); % If more than 1 S waves are after the first R wave and before the secnd R wave (rare), consider the one closest to the first R peak.
    end
    
    % T Wave.
    temp = idxs_t(idxs_t > idxs_r(1) & idxs_t < idxs_r(2));
    if isempty(temp)
        idxs_coherent_t(1) = nan;
        temp = [];
    else
        idxs_coherent_t(1) = temp(end); % If more than 1 T waves are after the first R wave and before the second R wave (rare), consider the one closest to the first R peak.
    end

    
    %% Cycle 2:End-1.
    for i = 2:length(idxs_r)-1
        
        % P Wave.
        temp = idxs_p(idxs_p > idxs_r(i-1) & idxs_p < idxs_r(i));
        if isempty(temp)
            idxs_coherent_p(i) = nan;
        else
            idxs_coherent_p(i) = temp(end); % If more than 1 P waves are detected before the current R wave and before the next R wave (rare), consider the one closest to the current R peak.
        end
        
        % Q Wave.
        temp = idxs_q(idxs_q > idxs_r(i-1) & idxs_q < idxs_r(i));
        if isempty(temp)
            idxs_coherent_q(i) = nan;
        else
            idxs_coherent_q(i) = temp(end); % If more than 1 P waves are detected before the current R wave and before the next R wave (rare), consider the one closest to the current R peak.
        end
        
        % R Wave.
        idxs_coherent_r(i) = idxs_r(i);
        
        % S Wave.
        temp = idxs_s(idxs_s > idxs_r(i) & idxs_s < idxs_r(i+1));
        if isempty(temp)
            idxs_coherent_s(i) = nan;
        else
            idxs_coherent_s(i) = temp(1); % If more than 1 S waves are detected after the current R wave and before the next R wave (rare), consider the one closest to the current R peak.
        end
        
        % T Wave.
        temp = idxs_t(idxs_t > idxs_r(i) & idxs_t < idxs_r(i+1));
        if isempty(temp)
            idxs_coherent_t(i) = nan;
        else
            idxs_coherent_t(i) = temp(1);  % If more than 1 S waves are detected after the current R wave and before the next R wave (rare), consider the one closest to the current R peak.
        end
    end
    

    %% Last Cycle.
    
    % P Wave.
    temp = idxs_p(idxs_p > idxs_r(end-1) & idxs_p < idxs_r(end));
    if isempty(temp) 
        idxs_coherent_p(end) = nan;
    else
        idxs_coherent_p(end) = temp(end); % If more than 1 P waves are detected before the last R wave (rare), consider the one closest to the last R peak.
    end
    
    % Q Wave.
    temp = idxs_q(idxs_q > idxs_r(end-1) & idxs_q < idxs_r(end));
    if isempty(temp) 
        idxs_coherent_q(end) = nan;
    else
        idxs_coherent_q(end) = temp(end); % If more than 1 Q waves are detected before the last R wave (rare), consider the one closest to the last R peak.
    end
    
    % R Wave.
    idxs_coherent_r(end) = idxs_r(end);
    
    % S Wave.
    temp = idxs_s(idxs_s > idxs_r(1) & idxs_s < idxs_r(2));
    if isempty(temp)
        idxs_coherent_s(end) = nan;
    else
        idxs_coherent_s(end) = temp(1); % If more than 1 S waves are detected before the last R wave (rare), consider the one closest to the last R peak.
    end
    
    % T Wave.
    temp = idxs_t(idxs_t > idxs_r(1) & idxs_t < idxs_r(2));
    if isempty(temp)
        idxs_coherent_t(end) = nan;
    else
        idxs_coherent_t(end) = temp(1); % If more than 1 T waves are detected before the last R wave (rare), consider the one closest to the last R peak.
    end
    

    %% Coherent Aggregation
    idxs_coherent_pqrst = [idxs_coherent_p, idxs_coherent_q, idxs_coherent_r, idxs_coherent_s, idxs_coherent_t];
    num_cycles = length(idxs_coherent_r);  
else
    idxs_coherent_pqrst = [];
    num_cycles = 0;
end
end

== matlab function FullCardioLabModel/SCG Analysis/Enabled SCG Analysis Subsystem/All Signals Signal Metric Characterization/SCG X Signal Metric Characterization/Average Signal-to-Noise Ratio Calculator/Average S1 Signal-to-Noise Ratio/Average S1 SNR Calculator ==
  data: fs input size=[1]; r_pos input; scg_signal input; average_s1_snr output size=[1]
function average_s1_snr = slk_average_s1snr_calculator(fs, r_pos, scg_signal)
% Function to calculate the average (mean) S1 signal-to-noise ratio from an SCG input signal, where:
% Signal = S1 complex
% Noise = rest of cycle

% The signal-to-noise ratio is considered to be the ratio of
% root-mean-square values of the signal and the noise.

if r_pos
    
    num_cycles = length(r_pos);
    
    s1snr = zeros(1,num_cycles); % Pre-initialization for speed.
    
    for i = 1:num_cycles - 1
        signal = scg_signal(r_pos(i):r_pos(i) + 0.2*fs); % The signal is the S1 complex.
        noise = scg_signal(r_pos(i) + 0.2*fs + 1:r_pos(i+1)); % The rest of the cycle is the noise.
        s1snr(i) = rms(signal)/rms(noise); % SnR is the ratio of rms(signal) to rms (noise).
    end
    
    average_s1_snr = mean(s1snr);
    
else
    
    average_s1_snr = nan;
   
end

== matlab function FullCardioLabModel/SCG Analysis/Enabled SCG Analysis Subsystem/All Signals Signal Metric Characterization/SCG X Signal Metric Characterization/Average Signal-to-Noise Ratio Calculator/Average S1X Signal-to-Noise Ratio/Average S1 SNR Amplitude Calculator ==
  data: fs input size=[1]; r_pos input; scg_signal input; average_s1x_snr output size=[1]
function average_s1x_snr = slk_average_s1xsnr_calculator(fs, r_pos, scg_signal)
% Function to calculate the average (mean) S1 signal-to-noise ratio from an SCG input signal, where:
% Signal = S1 complex
% Noise = rest of cycle EXCEPT the S2 complex

% The signal-to-noise ratio is considered to be the ratio of
% root-mean-square values of the signal and the noise.
    
num_cycles = length(r_pos);
s2_search_window_lims = [0.05*fs 0.3*fs]; % The window initially used to search for the S2 peak within the 'noise' segment.
s2_excise_window = fs*0.1; % The window length centered about the S2 peak (in samples) used to excise the S2 complex.

s1xsnr = zeros(1,num_cycles); % Pre-initialization for speed.

for i = 1:num_cycles - 1
    signal = scg_signal(r_pos(i):r_pos(i) + 0.2*fs); % The signal is the S1 complex.
 
    % Removing the S2 complex from the rest of the cycle.
    noise = scg_signal(1 + r_pos(i) + 0.2*fs:r_pos(i+1)); % Rest of the cycle.
    s2_search_window = noise(s2_search_window_lims(1):s2_search_window_lims(2)); % Defining the window where to search for the S2 peak.
    s2peak = s2_search_window_lims(1) + find(abs(s2_search_window) == max(abs(s2_search_window))); % Identifying the S2 peak within "noise".
    noise(s2peak(1) - s2_excise_window/2 : s2peak(1) + s2_excise_window/2) = []; % Removing the S2 complex.
    
    s1xsnr(i) = rms(signal)/rms(noise); % SnR is the ratio of rms(signal) to rms (noise).   
end

average_s1x_snr = mean(s1xsnr);

end

== matlab function FullCardioLabModel/SCG Analysis/Enabled SCG Analysis Subsystem/All Signals Signal Metric Characterization/SCG X Signal Metric Characterization/Average Signal-to-Noise Ratio Calculator/Average S2 Signal-to-Noise Ratio/Average S2 SNR Calculator ==
  data: fs input size=[1]; r_pos input; scg_signal input; average_s2_snr output size=[1]
function average_s2_snr = slk_average_s2snr_calculator(fs, r_pos, scg_signal)
% Function to calculate the average (mean) S2 signal-to-noise ratio from an SCG input signal, where:
% Signal = S2 complex
% Noise = rest of cycle (including the S1 complex)

% The signal-to-noise ratio is considered to be the ratio of root-mean-square values of the signal and the noise.
    
num_cycles = length(r_pos);
s2_search_window_lims = [0.25*fs 0.5*fs]; % The window initially used to search for the S2 peak within that cycle.
s2_identify_window = fs*0.15; % The window length centered about the S2 peak (in samples) used to identify the S2 complex.

s2_snr = zeros(1,num_cycles); % Pre-initialization for speed.

for i = 1:num_cycles - 1 % The last cycle isn't considered because there's a good chance it's cut off.
   
    cycle = scg_signal(r_pos(i):r_pos(i+1)); % The current heart cycle.

    s2_search_window = cycle(s2_search_window_lims(1):s2_search_window_lims(2)); % Defining the window where to search for the S2 peak.
    s2peak = s2_search_window_lims(1) + find(abs(s2_search_window)==max(abs(s2_search_window))); % Identifying the S2 peak within 'cycle'.
    
    signal = cycle(s2peak(1) - s2_identify_window/2 : s2peak(1) + s2_identify_window/2); % The S2 complex is the signal.
    noise = cycle;
    noise(s2peak(1) - s2_identify_window/2 : s2peak(1) + s2_identify_window/2)= []; % Defining the noise as everything except the S2 complex.

    s2_snr(i) = rms(signal)/rms(noise);
    
end

average_s2_snr = mean(s2_snr);

end

== matlab function FullCardioLabModel/SCG Analysis/Enabled SCG Analysis Subsystem/All Signals Signal Metric Characterization/SCG X Signal Metric Characterization/Average Signal-to-Noise Ratio Calculator/Average S2X Signal-to-Noise Ratio/Average S2X SNR Calculator ==
  data: fs input size=[1]; r_pos input; scg_signal input; average_s2x_snr output size=[1]
function average_s2x_snr = slk_average_s2xsnr_calculator(fs, r_pos, scg_signal)
% Function to calculate the average (mean) S2 signal-to-noise ratio from an SCG input signal, where:
% Signal = S2 complex
% Noise = rest of cycle EXCLUDING the S1 complex

% The signal-to-noise ratio is considered to be the ratio of root-mean-square values of the signal and the noise.
    
num_cycles = length(r_pos);
s1_excise_window_lims = [1 0.2*fs]; % The window used to excise the S1 complex from the noise.
s2_search_window_lims = [0.25*fs 0.5*fs]; % The window initially used to search for the S2 peak within that cycle.
s2_identify_window = fs*0.15; % The window length centered about the S2 peak (in samples) used to identify the S2 complex.

s2_snr = zeros(1,num_cycles); % Pre-initialization for speed.

for i = 1:num_cycles - 1
   
    cycle = scg_signal(r_pos(i):r_pos(i+1)); % The current heart cycle.

    s2_search_window = cycle(s2_search_window_lims(1):s2_search_window_lims(2)); % Defining the window where to search for the S2 peak.
    s2peak = s2_search_window_lims(1) + find(abs(s2_search_window) == max(abs(s2_search_window))); % Identifying the S2 peak within 'cycle'.
    
    signal = cycle(s2peak(1) - s2_identify_window/2 : s2peak(1) + s2_identify_window/2); % The S2 complex is the signal.
    noise = cycle;
    noise(s2peak(1) - s2_identify_window/2 : s2peak(1) + s2_identify_window/2)= []; % Removing the S2 complex from the noise.
    noise(s1_excise_window_lims(1):s1_excise_window_lims(2))= [];

    s2_snr(i) = rms(signal)/rms(noise);
    
end

average_s2x_snr = mean(s2_snr);

end
